simulink model "model_4"  (R2014a)
settings: Solver=ode3  StartTime=0.0  StopTime=30  FixedStep=0.1  RelTol=1e-3
settings Model: Creator=Павел  LastModifiedBy=Павел
settings DataIOCC: InspectSignalLogs=on

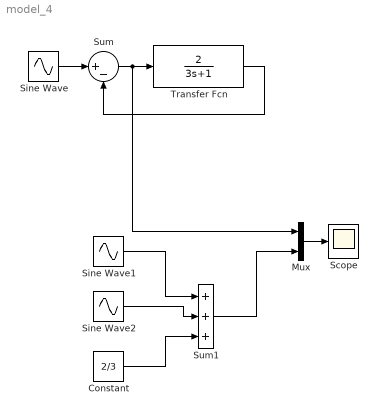
== system model_4 ==
  Constant : Constant  Value=2/3
  Mux : Mux  Inputs=2
  Scope : Scope
      settings: TimeRange=30  YMin=-1  YMax=2.5
  Sine Wave : Sin  Amplitude=3  Bias=2  Frequency=0.5  SampleTime=0
  Sine Wave1 : Sin  Frequency=0.5  Phase=90  SampleTime=0
  Sine Wave2 : Sin  Amplitude=1.8  Frequency=0.5  SampleTime=0
  Sum : Sum  Inputs=|+-
  Sum1 : Sum  Inputs=+++
  Transfer Fcn : TransferFcn  Numerator=[2]  Denominator=[3 1]
  wires:
  Sum/1 -> Mux/1, Transfer Fcn/1
  Transfer Fcn/1 -> Sum/2
  Sine Wave/1 -> Sum/1
  Sine Wave1/1 -> Sum1/1
  Sine Wave2/1 -> Sum1/2
  Constant/1 -> Sum1/3
  Mux/1 -> Scope/1
  Sum1/1 -> Mux/2
